simulink model "FullyControlledRectifier_updated"  (R2021a)
settings: Solver=VariableStepAuto  StartTime=0.0  StopTime=5  FixedStep=1e-6  RelTol=1e-3
values from neighbouring files (symbols this model uses):
  rated_load_torque = power_watt / rated_angular_speed    (= 20.3454584681)    [fully_controlled_rect_init_script.m]
libraries: spsThyristorLib x4, spsCurrentMeasurementLib x2, spsVoltageMeasurementLib x2, simulink_extras x2, spsMonostableLib x2, spsACVoltageSourceLib x1, spsDCMachineLib x1, spsDCVoltageSourceLib x1, spsGroundLib x1, spspowerguiLib x1
settings Model: Creator=dinesh  LastModifiedBy=USER
settings SolverCC: ZeroCrossAlgorithm=Adaptive  AlgebraicLoopSolver=TrustRegion
settings DataIOCC: ReturnWorkspaceOutputs=off
settings DebuggingCC: IgnoredZcDiagnostic=none  SFMachineParentedDataDiag=warning  ArithmeticOperatorsInVariantConditions=warning
settings SFSimCC: SimUseLocalCustomCode=off  CustomCodeUndefinedFunction=UseInterfaceOnly
settings RTWCC: RTWUseLocalCustomCode=off

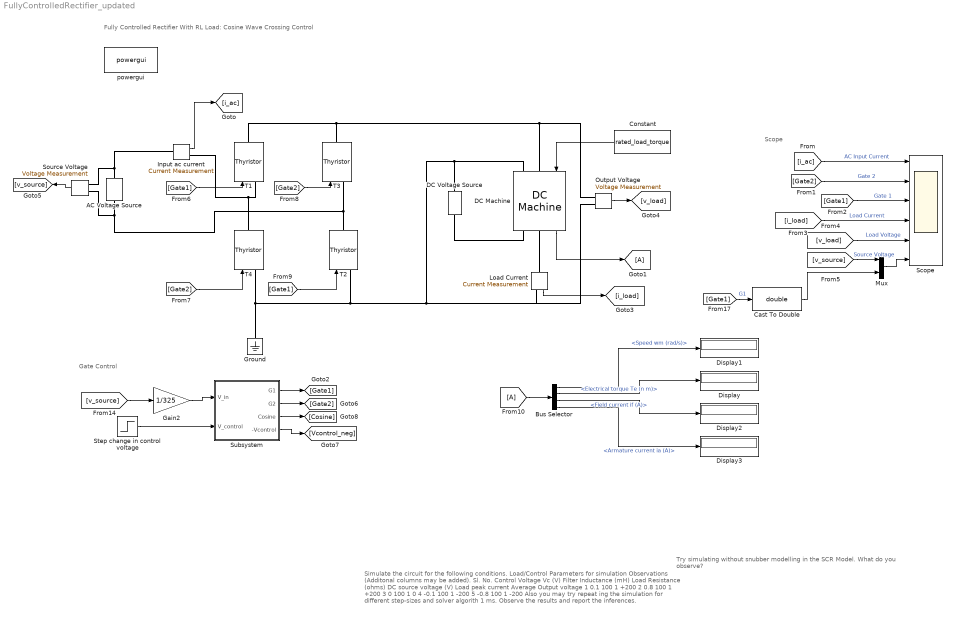
== system FullyControlledRectifier_updated ==
  note: Scope
  note: Gate Control
  note: Try simulating without snubber modelling in the SCR Model.
      | What do you observe?
  note: Fully Controlled Rectifier With RL Load: Cosine Wave Crossing Control
  note: Simulate the circuit for the following conditions.
      |
      | Load/Control Parameters for simulation
      | Observations (Additonal columns may be added).
      |
      | Sl. No.
      | Control Voltage Vc (V)
      | Filter Inductance (mH)
      | Load Resistance (ohms)
      | DC source voltage
      | (V)
      | Load peak current
      | Average Output voltage
      |
      | 1
      | 0.1
      | 100
      | 1
      | +200
      |
      | 2
      | 0.8
      | 100
      | 1
      | +200
      |
      | 3
      | 0
      | 100
      | 1
      | 0
      |
      | 4
      | -0.1
      | 100
      | 1
      | -200
      |
      | 5
      | -0.8
      | 100
      | 1
      | -200
      |
      | Also you may try repeat ing the simulation for different step-sizes and solver algorith 1 ms. Observe the results and report the inferences.
  AC Voltage Source : spsACVoltageSourceLib/AC Voltage Source  Amplitude=325  Phase=0  Frequency=50  SampleTime=0  Measurements=None  BusType=swing  Pref=10e3  Qref=0  Qmin=-inf  Qmax=+inf
  Bus Selector : BusSelector  OutputSignals=Speed wm (rad/s),Electrical torque Te (n m),Field current if (A),Armature current ia (A)
  Cast To Double : DataTypeConversion  OutDataTypeStr=double
  Constant : Constant  Value=rated_load_torque
  DC Machine : spsDCMachineLib/DC Machine  PresetModel=01: 5HP 240V 1750RPM Field:300V  MechanicalLoad=Torque TL  FieldType=Wound  ShowDetailedParameters=on  MeasurementBus=off  RLa=[2.581 0.028]  RLf=[281.2 156]  Laf=0.9483  MachineConstant=Torque constant (N.m/A)  Ke=1.8  Kt=1.8  J=0.02215  Bm=0.002953  Tf=0.5161  w0=1  Ifinit=-1.06685633001422  TsPowergui=0  TsBlock=-1
  DC Voltage Source : spsDCVoltageSourceLib/DC Voltage Source  Amplitude=300  Measurements=None
  Display{,1..3} (4 alike) : Display
  Gain2 : Gain  Gain=1/325
  Ground : spsGroundLib/Ground  LConnTagsString=a
  Input ac current : spsCurrentMeasurementLib/Current Measurement  PhasorSimulation=off  OutputType=Complex  PSBequivalent=0
  Load Current : spsCurrentMeasurementLib/Current Measurement  PhasorSimulation=off  OutputType=Complex  PSBequivalent=0
  Mux : Mux  Inputs=2
  Output Voltage : spsVoltageMeasurementLib/Voltage Measurement  PhasorSimulation=off  OutputType=Complex  PSBequivalent=0
  Scope : Scope  NumInputPorts=6
  Source Voltage : spsVoltageMeasurementLib/Voltage Measurement  PhasorSimulation=off  OutputType=Complex  PSBequivalent=0
  Step change in control voltage : Step  Time=2  Before=-0.1  After=-0.8  SampleTime=0
  Subsystem : Subsystem
  T1 : spsThyristorLib/Thyristor  Ron=0.001  Lon=0  Vf=0.8  IC=0  Rs=inf  Cs=0.22e-6  Measurements=off
  T2 : spsThyristorLib/Thyristor  Ron=0.001  Lon=0  Vf=0.8  IC=0  Rs=inf  Cs=0.22e-6  Measurements=off
  T3 : spsThyristorLib/Thyristor  Ron=0.001  Lon=0  Vf=0.8  IC=0  Rs=inf  Cs=inf  Measurements=off
  T4 : spsThyristorLib/Thyristor  Ron=0.001  Lon=0  Vf=0.8  IC=0  Rs=inf  Cs=0.22e-6  Measurements=off
  powergui : spspowerguiLib/powergui  Priority=1  SimulationMode=Continuous  SampleTime=50e-6  frequency=60  Iterations=50  frequencyindice=50  Pbase=100e6  ErrMax=1e-4  UnitsV=kV  UnitsW=MW  buscounter=0  FunctionMessages=off  echomessages=off  EnableUseOfTLC=off  CurrentSourceSwitches=off  DisableSnubberDevices=off  DisableRonSwitches=off  DisableVfSwitches=off  DisplayEquations=off  AutomaticDiscreteSolvers=off  SolverType=Tustin/Backward Euler (TBE)  Interpol=off  ExternalGateDelay=off  methode=off  Ts=100  x0status=blocks  SPID=off  SwTol=0  HookPort=off  NonlinearTolerance=1e-4  nMaxIteration=100  ContinueOnMaxIteration=off  RestoreLinks=warning  ResistiveCurrentMeasurement=off  Frange=[0:2:500]  Ylog=off  Xlog=on  ShowGrid=off  save=off  variable=ZData  structure=0  ZoomFFT=off  StartTime=0.0  cycles=1  DisplayStyle=1  fundamental=60  FreqAxis=off  MaxFrequency=1000  frequencyindicesteady=1  RmsSteady=1  display=off
  wires:
  Input ac current/1 -> [i_ac]
  Load Current/1 -> [i_load]
  Output Voltage/1 -> [v_load]
  Source Voltage/1 -> [v_source]
  [Gate1] -> T1/1
  [Gate2] -> T4/1
  [Gate2] -> T3/1
  [Gate1] -> T2/1
  [v_source] -> Gain2/1
  Subsystem/1(G1) -> [Gate1]
  Gain2/1 -> Subsystem/1(V_in)
  Subsystem/2(G2) -> [Gate2]
  Subsystem/3(Cosine) -> [Cosine]
  Subsystem/4(-Vcontrol) -> [Vcontrol_neg]
  [v_load] -> Scope/5  "Load Voltage"
  [Gate1] -> Scope/3  "Gate 1"
  [i_ac] -> Scope/1  "AC Input Current"
  [i_load] -> Scope/4  "Load Current"
  [Gate2] -> Scope/2  "Gate 2"
  [v_source] -> Mux/1  "Source Voltage"
  Mux/1 -> Scope/6
  [Gate1] -> Cast To Double/1  "G1"
  Cast To Double/1 -> Mux/2
  Step change in control voltage/1 -> Subsystem/2(V_control)
  Constant/1 -> DC Machine/1
  DC Machine/1 -> [A]
  [A] -> Bus Selector/1
  Bus Selector/2 -> Display/1  "<Electrical torque Te (n m)>"
  Bus Selector/1 -> Display1/1  "<Speed wm (rad/s)>"
  Bus Selector/3 -> Display2/1  "<Field current if (A)>"
  Bus Selector/4 -> Display3/1  "<Armature current ia (A)>"
  connections:
  AC Voltage Source/RConn1 -- Input ac current/LConn1 -- Source Voltage/LConn1
  Input ac current/RConn1 -- T1/LConn1 -- T4/RConn1
  DC Voltage Source/LConn1 -- T4/LConn1 -- Ground/LConn1 -- T2/LConn1 -- Load Current/RConn1 -- Output Voltage/LConn2 -- DC Machine/LConn2
  AC Voltage Source/LConn1 -- T2/RConn1 -- T3/LConn1 -- Source Voltage/LConn2
  T1/RConn1 -- DC Machine/LConn1 -- Output Voltage/LConn1 -- T3/RConn1
  Load Current/LConn1 -- DC Machine/RConn1
  DC Voltage Source/RConn1 -- DC Machine/RConn2

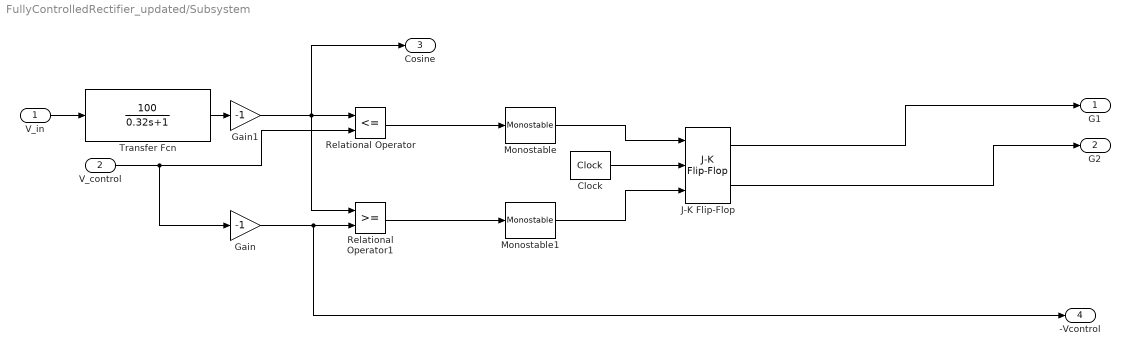
== system FullyControlledRectifier_updated/Subsystem ==
  V_in : Inport
  V_control : Inport  Port=2
  Clock : simulink_extras/Flip Flops/Clock  period=100e-6
  Gain : Gain  Gain=-1
  Gain1 : Gain  Gain=-1
  J-K Flip-Flop : simulink_extras/Flip Flops/J-K Flip-Flop  initial_condition=0
  Monostable : spsMonostableLib/Monostable  EdgeDetect=Rising  PulseDuration=1e-3  ic=0  Ts=0
      settings: SourceProductBaseCode=PS
  Monostable1 : spsMonostableLib/Monostable  EdgeDetect=Rising  PulseDuration=1e-3  ic=0  Ts=0
      settings: SourceProductBaseCode=PS
  Relational Operator : RelationalOperator  Operator=<=  OutDataTypeStr=boolean  RndMeth=Simplest
  Relational Operator1 : RelationalOperator  OutDataTypeStr=boolean  RndMeth=Simplest
  Transfer Fcn : TransferFcn  Numerator=[100]  Denominator=[0.32 1]
  G1 : Outport  VectorParamsAs1DForOutWhenUnconnected=off
  G2 : Outport  Port=2  VectorParamsAs1DForOutWhenUnconnected=off
  Cosine : Outport  Port=3  VectorParamsAs1DForOutWhenUnconnected=off
  -Vcontrol : Outport  Port=4  VectorParamsAs1DForOutWhenUnconnected=off
  wires:
  Transfer Fcn/1 -> Gain1/1
  V_control/1 -> Relational Operator/2, Gain/1
  Gain/1 -> -Vcontrol/1, Relational Operator1/2
  Relational Operator/1 -> Monostable/1
  Relational Operator1/1 -> Monostable1/1
  V_in/1 -> Transfer Fcn/1
  Monostable/1 -> J-K Flip-Flop/1
  Monostable1/1 -> J-K Flip-Flop/3
  J-K Flip-Flop/1 -> G1/1
  J-K Flip-Flop/2 -> G2/1
  Clock/1 -> J-K Flip-Flop/2
  Gain1/1 -> Cosine/1, Relational Operator1/1, Relational Operator/1
